simulink model "IM_VF_SVM"  (R2014a)
settings: Solver=ode23tb  StartTime=0.0  StopTime=1  RelTol=1e-3
libraries: powerlib x7, simulink x1
settings Model: Creator=ninad gaikawad  LastModifiedBy=ninad gaikawad
settings SolverCC: ZeroCrossAlgorithm=Adaptive

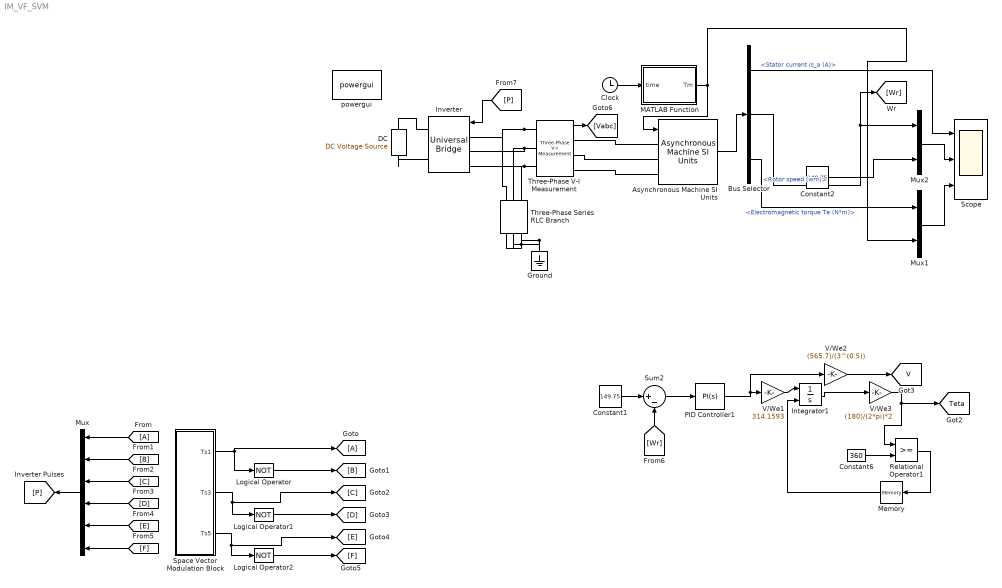
== system IM_VF_SVM ==
  Asynchronous Machine SI Units : powerlib/Machines/Asynchronous Machine SI Units  PresetModel="15:  5.4 HP (4KW)   400 V  50Hz 1430 RPM"  MechanicalLoad=Torque Tm  ShowDetailedParameters=on  RotorType=Squirrel-cage  ReferenceFrame=Rotor  Units=SI  MeasurementBus=off  NominalParameters=[4000 400 50]  Stator=[1.405 0.005839]  Rotor=[1.395 0.005839]  Cage1=[ 0.022 0.226/377]  Cage2=[ 0.022 0.226/377]  Lm=0.1722  Mechanical=[0.0131 0.002985 2]  PolePairs=2  InitialConditions=[1 0 0 0 0 0 0 0]  SimulateSaturation=off  Saturation=[14.03593122, 27.81365428, 53.79336849, 72.68890987, 97.98006896, 148.6815601, 215.7428561, 302.9841135, 420.4778367 ; 230, 322, 414, 460, 506, 552, 598, 644, 690]  LoadFlowParameters=1492000  TsPowergui=0  TsBlock=-1  IterativeModel=Trapezoidal non iterative  Pmec=0
  Bus Selector : BusSelector  OutputSignals=Stator measurements.Stator current is_a (A),Mechanical.Rotor speed (wm),Mechanical.Electromagnetic torque Te (N*m)
  Clock : Clock
  Constant1 : Constant  Value=149.75
  Constant2 : Constant  Value=149.75
  Constant6 : Constant  Value=360
  "DC " : powerlib/Electrical Sources/DC Voltage Source  Amplitude=565.7  Measurements=None
  Ground : powerlib/Elements/Ground  LConnTagsString=a
  Integrator1 : Integrator  ExternalReset=rising
  Inverter : powerlib/Power Electronics/Universal Bridge  Arms=3  SnubberResistance=1e5  SnubberCapacitance=inf  Device=IGBT / Diodes  Ron=1e-3  Lon=0  ForwardVoltages="[  0  0  ]"  ForwardVoltage=0  GTOparameters=[ 10e-6 , 20e-6 ]  IGBTparameters=[ 1e-6 , 2e-6 ]  Measurements=None  Measurements_2=None  converterType=Rectifier
  Logical Operator : Logic  Operator=NOT  AllPortsSameDT=off  OutDataTypeStr=boolean
  Logical Operator1 : Logic  Operator=NOT  AllPortsSameDT=off  OutDataTypeStr=boolean
  Logical Operator2 : Logic  Operator=NOT  AllPortsSameDT=off  OutDataTypeStr=boolean
  MATLAB Function : MATLAB Function  TreatAsAtomicUnit=on
  Memory : Memory
  Mux : Mux  Inputs=6
  Mux1 : Mux  Inputs=2
  Mux2 : Mux  Inputs=2
  PID Controller1 : simulink/Continuous/PID Controller  Controller=PI  TimeDomain=Continuous-time  SampleTime=1  IntegratorMethod=Forward Euler  FilterMethod=Forward Euler  Form=Parallel  P=0.001  I=0.01  D=0  N=100  InitialConditionSource=internal  InitialConditionForIntegrator=0  InitialConditionForFilter=0  ExternalReset=none  LimitOutput=on  UpperSaturationLimit=0.99  LowerSaturationLimit=0  LinearizeAsGain=on  AntiWindupMode=clamping  Kb=1  TrackingMode=off  Kt=1  PParamMin=[]  PParamMax=[]  IParamMin=[]  IParamMax=[]  DParamMin=[]  DParamMax=[]  NParamMin=[]  NParamMax=[]  KbParamMin=[]  KbParamMax=[]  KtParamMin=[]  KtParamMax=[]  POutMin=[]  POutMax=[]  IOutMin=[]  IOutMax=[]  DOutMin=[]  DOutMax=[]  NOutMin=[]  NOutMax=[]  KbOutMin=[]  KbOutMax=[]  KtOutMin=[]  KtOutMax=[]  IntegratorOutMin=[]  IntegratorOutMax=[]  FilterOutMin=[]  FilterOutMax=[]  SumOutMin=[]  SumOutMax=[]  SumI1OutMin=[]  SumI1OutMax=[]  SumI2OutMin=[]  SumI2OutMax=[]  SumI3OutMin=[]  SumI3OutMax=[]  SumDOutMin=[]  SumDOutMax=[]  SaturationOutMin=[]  SaturationOutMax=[]  IntegratorContinuousStateAttributes=''  IntegratorStateMustResolveToSignalObject=off  IntegratorRTWStateStorageClass=Auto  FilterContinuousStateAttributes=''  FilterStateMustResolveToSignalObject=off  FilterRTWStateStorageClass=Auto
  Relational Operator1 : RelationalOperator  OutDataTypeStr=boolean
  Scope : Scope  NumInputPorts=3
      settings: YMin=-5~-5~-5  YMax=5~5~5
  Space Vector Modulation Block : Subsystem
  Sum2 : Sum  Inputs=|+-
  Three-Phase Series RLC Branch : powerlib/Elements/Three-Phase Series RLC Branch  LConnTagsString=A|B|C  RConnTagsString=A|B|C  BranchType=R  Resistance=1e6  Inductance=1e-3  Capacitance=1e-6  Measurements=None
  Three-Phase V-I Measurement : powerlib/Measurements/Three-Phase V-I Measurement  VoltageMeasurement=phase-to-phase  SetLabelV=off  LabelV=Vabc  Vpu=off  VpuLL=off  CurrentMeasurement=no  SetLabelI=off  LabelI=Iabc  Ipu=off  Pbase=100e6  Vbase=500e3  OutputType=Complex  PhasorSimulation=off  PSBequivalent=0
  V/We1 : Gain  Gain=314.1593
  V/We2 : Gain  Gain=(565.7)/(3^(0.5))
  V/We3 : Gain  Gain=(180)/(2*pi)*2
  powergui : powerlib/powergui  Priority=1  SimulationMode=Continuous  SolverType=Tustin  SampleTime=50e-6  frequency=60  SPID=off  DisableSnubberDevices=off  DisableRonSwitches=off  DisableVfSwitches=off  SwTol=0  Interpol=off  DisplayEquations=off  Ts=0  methode=off  frequencyindice=50  Pbase=100e6  ErrMax=1e-4  Iterations=50  UnitsV=kV  UnitsW=MW  FunctionMessages=off  echomessages=off  HookPort=off  EnableUseOfTLC=off  x0status=blocks  RestoreLinks=warning  ResistiveCurrentMeasurement=off  Frange=[0:2:500]  Ylog=off  Xlog=on  ShowGrid=off  save=off  variable=ZData  structure=0  ZoomFFT=off  StartTime=0.0  cycles=1  DisplayStyle=1  fundamental=60  FreqAxis=off  MaxFrequency=1000  frequencyindicesteady=1  RmsSteady=1  display=off
  tag scope: Teta=global, V=global
  wires:
  Space Vector Modulation Block/1(Ts1) -> Logical Operator/1, [A]
  Space Vector Modulation Block/2(Ts3) -> [C], Logical Operator1/1
  Space Vector Modulation Block/3(Ts5) -> [E], Logical Operator2/1
  Logical Operator/1 -> [B]
  Logical Operator1/1 -> [D]
  Logical Operator2/1 -> [F]
  [A] -> Mux/1
  [B] -> Mux/2
  [C] -> Mux/3
  [D] -> Mux/4
  [E] -> Mux/5
  [F] -> Mux/6
  Asynchronous Machine SI Units/1 -> Bus Selector/1
  Mux1/1 -> Scope/3
  Mux2/1 -> Scope/2
  [P] -> Inverter/1
  Three-Phase V-I Measurement/1 -> [Vabc]
  Bus Selector/1 -> Scope/1  "<Stator current is_a (A)>"
  Bus Selector/2 -> Mux2/1, [Wr]  "<Rotor speed (wm)>"
  Bus Selector/3 -> Mux1/1  "<Electromagnetic torque Te (N*m)>"
  Constant2/1 -> Mux2/2
  Constant1/1 -> Sum2/1
  V/We1/1 -> Integrator1/1
  PID Controller1/1 -> V/We2/1, V/We1/1
  Clock/1 -> MATLAB Function/1(time)
  MATLAB Function/1(Tm) -> Asynchronous Machine SI Units/1, Mux1/2
  [Wr] -> Sum2/2
  Sum2/1 -> PID Controller1/1
  Mux/1 -> [P]
  Constant6/1 -> Relational Operator1/2
  V/We3/1 -> [Teta], Relational Operator1/1
  Relational Operator1/1 -> Memory/1
  Integrator1/1 -> V/We3/1
  V/We2/1 -> [V]
  Memory/1 -> Integrator1/2
  connections:
  Three-Phase V-I Measurement/LConn2 -- Inverter/LConn2 -- Three-Phase Series RLC Branch/LConn2
  Three-Phase V-I Measurement/LConn1 -- Inverter/LConn1 -- Three-Phase Series RLC Branch/LConn1
  Three-Phase V-I Measurement/LConn3 -- Inverter/LConn3 -- Three-Phase Series RLC Branch/LConn3
  Ground/LConn1 -- Three-Phase Series RLC Branch/RConn3 -- Three-Phase Series RLC Branch/RConn1 -- Three-Phase Series RLC Branch/RConn2
  "DC "/LConn1 -- Inverter/RConn2
  Three-Phase V-I Measurement/RConn3 -- Asynchronous Machine SI Units/LConn3
  Three-Phase V-I Measurement/RConn2 -- Asynchronous Machine SI Units/LConn2
  "DC "/RConn1 -- Inverter/RConn1
  Three-Phase V-I Measurement/RConn1 -- Asynchronous Machine SI Units/LConn1

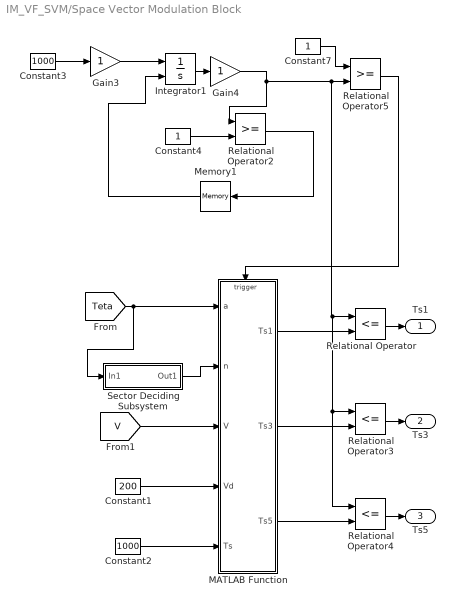
== system IM_VF_SVM/Space Vector Modulation Block ==
  Constant1 : Constant  Value=200
  Constant2 : Constant  Value=1000
  Constant3 : Constant  Value=1000
  Constant4 : Constant
  Constant7 : Constant
  Gain3 : Gain
  Gain4 : Gain
  Integrator1 : Integrator  ExternalReset=rising
  MATLAB Function : MATLAB Function  TreatAsAtomicUnit=on
  Memory1 : Memory
  Relational Operator : RelationalOperator  Operator=<=  OutDataTypeStr=boolean
  Relational Operator2 : RelationalOperator  OutDataTypeStr=boolean
  Relational Operator3 : RelationalOperator  Operator=<=  OutDataTypeStr=boolean
  Relational Operator4 : RelationalOperator  Operator=<=  OutDataTypeStr=boolean
  Relational Operator5 : RelationalOperator  OutDataTypeStr=boolean
  Sector Deciding Subsystem : Subsystem
  Ts1 : Outport
  Ts3 : Outport  Port=2
  Ts5 : Outport  Port=3
  wires:
  Constant1/1 -> MATLAB Function/4(Vd)
  [V] -> MATLAB Function/3(V)
  Sector Deciding Subsystem/1(Out1) -> MATLAB Function/2(n)
  Gain3/1 -> Integrator1/1
  Gain4/1 -> Relational Operator4/1, Relational Operator3/1, Relational Operator/1, Relational Operator5/2, Relational Operator2/1
  Relational Operator2/1 -> Memory1/1
  Constant3/1 -> Gain3/1
  Integrator1/1 -> Gain4/1
  Constant4/1 -> Relational Operator2/2
  Constant2/1 -> MATLAB Function/5(Ts)
  MATLAB Function/3(Ts5) -> Relational Operator4/2
  Relational Operator4/1 -> Ts5/1
  Relational Operator/1 -> Ts1/1
  Relational Operator3/1 -> Ts3/1
  MATLAB Function/2(Ts3) -> Relational Operator3/2
  MATLAB Function/1(Ts1) -> Relational Operator/2
  Constant7/1 -> Relational Operator5/1
  Relational Operator5/1 -> MATLAB Function/Trigger
  Memory1/1 -> Integrator1/2
  [Teta] -> Sector Deciding Subsystem/1(In1), MATLAB Function/1(a)

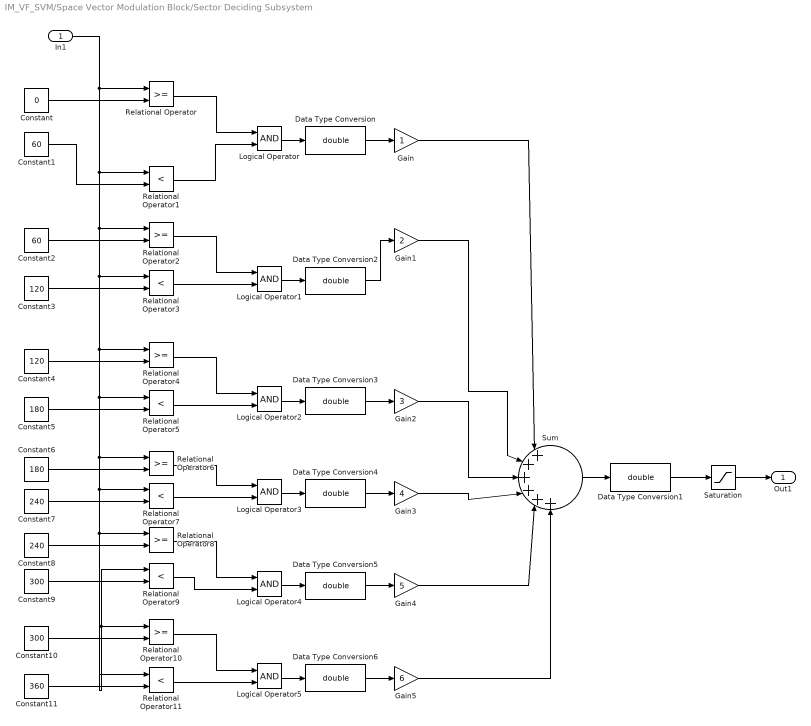
== system IM_VF_SVM/Space Vector Modulation Block/Sector Deciding Subsystem ==
  In1 : Inport
  Constant : Constant  Value=0
  Constant1 : Constant  Value=60
  Constant10 : Constant  Value=300
  Constant11 : Constant  Value=360
  Constant2 : Constant  Value=60
  Constant3 : Constant  Value=120
  Constant4 : Constant  Value=120
  Constant5 : Constant  Value=180
  Constant6 : Constant  Value=180
  Constant7 : Constant  Value=240
  Constant8 : Constant  Value=240
  Constant9 : Constant  Value=300
  Data Type Conversion{,1..6} (7 alike) : DataTypeConversion  OutDataTypeStr=double
  Gain : Gain
  Gain1 : Gain  Gain=2
  Gain2 : Gain  Gain=3
  Gain3 : Gain  Gain=4
  Gain4 : Gain  Gain=5
  Gain5 : Gain  Gain=6
  Logical Operator{,1..5} (6 alike) : Logic  AllPortsSameDT=off  OutDataTypeStr=boolean
  Relational Operator{,2,4,6,8,10} (6 alike) : RelationalOperator  OutDataTypeStr=boolean
  Relational Operator{1,3,5,7,9,11} (6 alike) : RelationalOperator  Operator=<  OutDataTypeStr=boolean
  Saturation : Saturate  UpperLimit=6  LowerLimit=1
  Sum : Sum  Inputs=|++++++
  Out1 : Outport
  wires:
  Constant1/1 -> Relational Operator1/2
  Constant/1 -> Relational Operator/2
  Relational Operator1/1 -> Logical Operator/2
  Relational Operator/1 -> Logical Operator/1
  Logical Operator/1 -> Data Type Conversion/1
  Data Type Conversion/1 -> Gain/1
  Gain/1 -> Sum/1
  Sum/1 -> Data Type Conversion1/1
  Data Type Conversion1/1 -> Saturation/1
  Saturation/1 -> Out1/1
  Constant3/1 -> Relational Operator3/2
  Constant2/1 -> Relational Operator2/2
  Relational Operator3/1 -> Logical Operator1/2
  Relational Operator2/1 -> Logical Operator1/1
  Logical Operator1/1 -> Data Type Conversion2/1
  Data Type Conversion2/1 -> Gain1/1
  Gain1/1 -> Sum/2
  Constant5/1 -> Relational Operator5/2
  Constant4/1 -> Relational Operator4/2
  Relational Operator5/1 -> Logical Operator2/2
  Relational Operator4/1 -> Logical Operator2/1
  Logical Operator2/1 -> Data Type Conversion3/1
  Data Type Conversion3/1 -> Gain2/1
  Gain2/1 -> Sum/3
  Constant7/1 -> Relational Operator7/2
  Constant6/1 -> Relational Operator6/2
  Relational Operator7/1 -> Logical Operator3/2
  Relational Operator6/1 -> Logical Operator3/1
  Logical Operator3/1 -> Data Type Conversion4/1
  Data Type Conversion4/1 -> Gain3/1
  Constant9/1 -> Relational Operator9/2
  Constant8/1 -> Relational Operator8/2
  Relational Operator9/1 -> Logical Operator4/2
  Relational Operator8/1 -> Logical Operator4/1
  Logical Operator4/1 -> Data Type Conversion5/1
  Data Type Conversion5/1 -> Gain4/1
  Gain4/1 -> Sum/5
  Constant11/1 -> Relational Operator11/2
  Constant10/1 -> Relational Operator10/2
  In1/1 -> Relational Operator4/1, Relational Operator9/1, Relational Operator11/1, Relational Operator10/1, Relational Operator8/1, Relational Operator7/1, Relational Operator6/1, Relational Operator5/1, Relational Operator3/1, Relational Operator2/1, Relational Operator1/1, Relational Operator/1
  Relational Operator11/1 -> Logical Operator5/2
  Relational Operator10/1 -> Logical Operator5/1
  Logical Operator5/1 -> Data Type Conversion6/1
  Data Type Conversion6/1 -> Gain5/1
  Gain5/1 -> Sum/6
  Gain3/1 -> Sum/4

== matlab function IM_VF_SVM/MATLAB Function ==
  data: Tm output; time input
function Tm = mechanical_torque(time)

if (time < 0.4 || time > 0.6)
Tm = 0;
else
Tm = 26.71;
end
end

== matlab function IM_VF_SVM/Space Vector Modulation Block/MATLAB Function ==
  data: a input; Ts1 output; Ts3 output; n input; V input; Vd input; Ts input; Ts5 output
  events: trigger input RISING_EDGE_EVENT
function [Ts1,Ts3,Ts5] = fcn(a,n,V,Vd,Ts)

a=a.*pi./180;
s=(3.^0.5).*(V/Vd).*Ts;
Ta=s.*sin((n.*pi./3)-a);
Tb=s.*sin(a-(n-1).*pi./3);
To=Ts-Ta-Tb;
Ts1=0;Ts3=0;Ts5=0;
switch n
    case 1
        Ts1=(Ts-(Ta+Tb+To./2))./Ts;
        Ts3=(Ts-(Tb+To./2))./Ts;
        Ts5=(Ts-(To./2))./Ts;
    case 2
        Ts1=(Ts-(Ta+To./2))./Ts;
        Ts3=(Ts-(Ta+Tb+To./2))./Ts;
        Ts5=(Ts-(To./2))./Ts;
    case 3
        Ts1=(Ts-(To./2))./Ts;
        Ts3=(Ts-(Ta+Tb+To./2))./Ts;
        Ts5=(Ts-(Tb+To./2))./Ts;
    case 4
        Ts1=(Ts-(To./2))./Ts;
        Ts3=(Ts-(Ta+To./2))./Ts;
        Ts5=(Ts-(Ta+Tb+To./2))./Ts;
    case 5
        Ts1=(Ts-(Tb+To./2))./Ts;
        Ts3=(Ts-(To./2))./Ts;
        Ts5=(Ts-(Ta+Tb+To./2))./Ts;
    case 6
        Ts1=(Ts-(Ta+Tb+To./2))./Ts;
        Ts3=(Ts-(To./2))./Ts;
        Ts5=(Ts-(Ta+To./2))./Ts;
end
return;
